simulink model "MPCSimulink"  (R2023b)
settings: Solver=VariableStepAuto  StartTime=0.0  StopTime=Tsim  RelTol=1e-3
undefined symbols (not defined in the file): distFinalValue, distInitialValue, KE, KF, Kr, noiseFinalValue, noiseInitialValue, refFinalValue, refInitialValue, ssA, ssB, ssD, ssH, Tdist, Tnoise, Tref, Ts
libraries: cstblocks x2
settings Model: Creator=klysm  LastModifiedBy=klysm

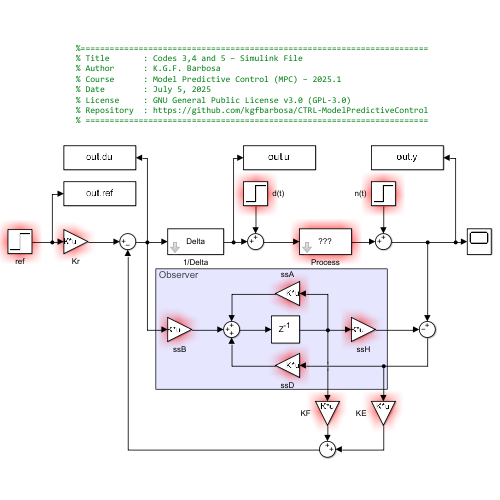
[thumbnail: Simulink's stored preview of the top-level diagram]
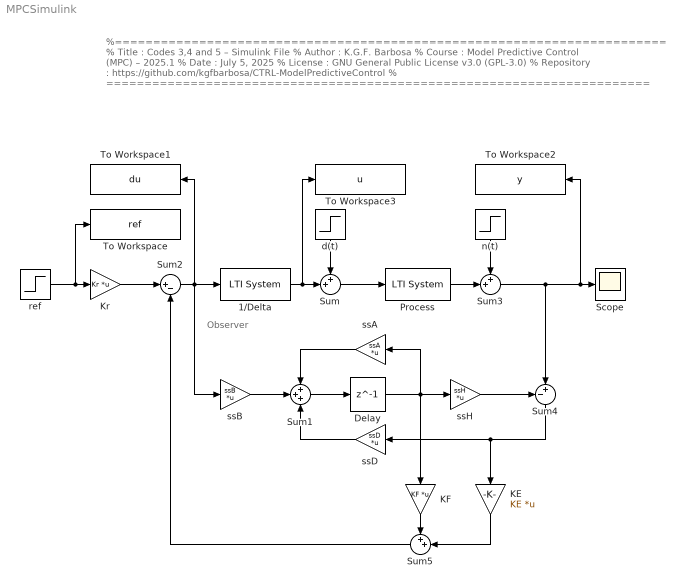
== system MPCSimulink ==
  note: %========================================================================
      | % Title : Codes 3,4 and 5 – Simulink File
      | % Author : K.G.F. Barbosa
      | % Course : Model Predictive Control (MPC) – 2025.1
      | % Date : July 5, 2025
      | % License : GNU General Public License v3.0 (GPL-3.0)
      | % Repository : https://github.com/kgfbarbosa/CTRL-ModelPredictiveControl
      | % =======================================================================
  note: Observer
  1/Delta : cstblocks/LTI System  sys=Delta  IC=[]  PadeOrder=0
  Delay : Delay  DelayLength=1  SampleTime=Ts
  KE : Gain  Gain=KE  Multiplication=Matrix(K*u)
  KF : Gain  Gain=KF  Multiplication=Matrix(K*u)
  Kr : Gain  Gain=Kr  Multiplication=Matrix(K*u)
  Process : cstblocks/LTI System  sys=Gz  IC=[]  PadeOrder=0
  Scope : Scope
  Sum : Sum  Inputs=++|
  Sum1 : Sum  Inputs=+++
  Sum2 : Sum  Inputs=|+-
  Sum3 : Sum  Inputs=++|
  Sum4 : Sum  Inputs=-+|
  Sum5 : Sum  Inputs=++|
  To Workspace : ToWorkspace  VariableName=ref  SampleTime=Ts
  To Workspace1 : ToWorkspace  VariableName=du  SampleTime=Ts
  To Workspace2 : ToWorkspace  VariableName=y  SampleTime=Ts
  To Workspace3 : ToWorkspace  VariableName=u  SampleTime=Ts
  d(t) : Step  Time=Tdist  Before=distInitialValue  After=distFinalValue  SampleTime=Ts
  n(t) : Step  Time=Tnoise  Before=noiseInitialValue  After=noiseFinalValue  SampleTime=Ts
  ref : Step  Time=Tref  Before=refInitialValue  After=refFinalValue  SampleTime=Ts
  ssA : Gain  Gain=ssA  Multiplication=Matrix(K*u)
  ssB : Gain  Gain=ssB  Multiplication=Matrix(K*u)
  ssD : Gain  Gain=ssD  Multiplication=Matrix(K*u)
  ssH : Gain  Gain=ssH  Multiplication=Matrix(K*u)
  wires:
  ref/1 -> To Workspace/1, Kr/1
  Sum2/1 -> 1/Delta/1, ssB/1, To Workspace1/1
  Kr/1 -> Sum2/1
  1/Delta/1 -> To Workspace3/1, Sum/2
  Sum/1 -> Process/1
  Process/1 -> Sum3/2
  ssB/1 -> Sum1/2
  ssA/1 -> Sum1/1
  Sum3/1 -> Sum4/2, To Workspace2/1, Scope/1
  Delay/1 -> ssA/1, KF/1, ssH/1
  Sum1/1 -> Delay/1
  Sum4/1 -> ssD/1, KE/1
  ssD/1 -> Sum1/3
  ssH/1 -> Sum4/1
  KF/1 -> Sum5/1
  KE/1 -> Sum5/2
  Sum5/1 -> Sum2/2
  d(t)/1 -> Sum/1
  n(t)/1 -> Sum3/1
